simulink model "Sistema_Seguimiento_Tipo1_Con_Planta_Tipo_1_Sin_Matrices"  (R2016a)
settings: Solver=VariableStepAuto  StartTime=0.0  StopTime=10.0  RelTol=1e-3
settings Model: Creator=Abel  LastModifiedBy=Abel

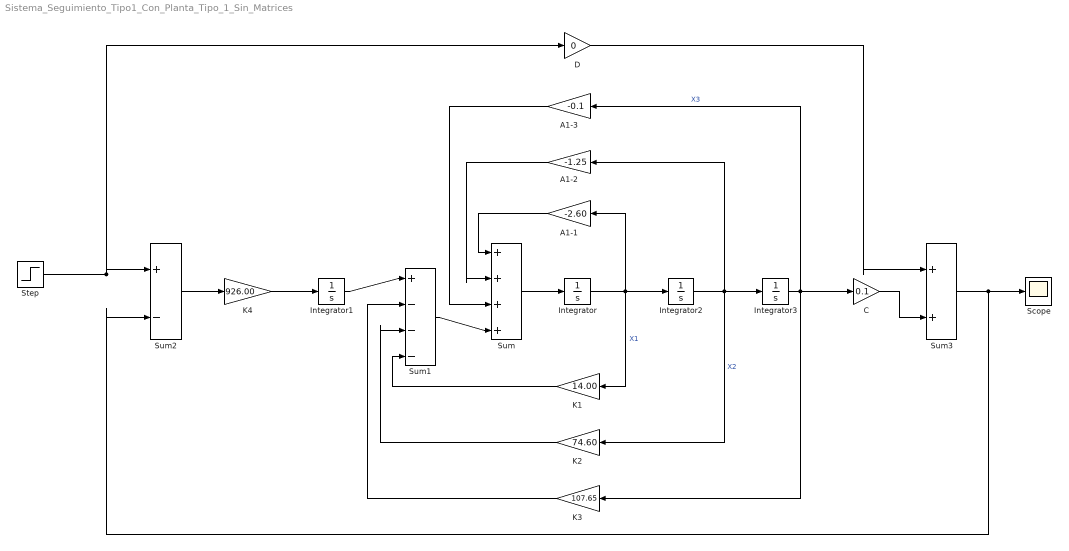
== system Sistema_Seguimiento_Tipo1_Con_Planta_Tipo_1_Sin_Matrices ==
  A1-1 : Gain  Gain=-2.60
  A1-2 : Gain  Gain=-1.25
  A1-3 : Gain  Gain=-0.1
  C : Gain  Gain=0.1
  D : Gain  Gain=0
  Integrator{,1..3} (4 alike) : Integrator
  K1 : Gain  Gain=14.00
  K2 : Gain  Gain=74.60
  K3 : Gain  Gain=107.65
  K4 : Gain  Gain=926.00
  Scope : Scope
  Step : Step  SampleTime=0
  Sum : Sum  Inputs=|+|+|+|+|
  Sum1 : Sum  Inputs=|+|-|-|-|
  Sum2 : Sum  Inputs=|+|-|
  Sum3 : Sum  Inputs=|+|+|
  wires:
  Integrator/1 -> K1/1, A1-1/1, Integrator2/1  "X1"
  Integrator2/1 -> K2/1, A1-2/1, Integrator3/1  "X2"
  Sum/1 -> Integrator/1
  A1-1/1 -> Sum/1
  A1-2/1 -> Sum/2
  A1-3/1 -> Sum/3
  Integrator3/1 -> C/1, K3/1, A1-3/1  "X3"
  Sum1/1 -> Sum/4
  K1/1 -> Sum1/4
  K2/1 -> Sum1/3
  K3/1 -> Sum1/2
  Integrator1/1 -> Sum1/1
  K4/1 -> Integrator1/1
  Sum2/1 -> K4/1
  Step/1 -> D/1, Sum2/1
  C/1 -> Sum3/2
  D/1 -> Sum3/1
  Sum3/1 -> Sum2/2, Scope/1
